simulink model "ALFlight3"  (R2019a)
settings: Solver=VariableStepAuto  StartTime=0.0  StopTime=100  RelTol=1e-3
InitFcn:
  | Ts=.05
  | load('goodMPC.mat')
  | %load('fault2mpc.mat')
  | global counts
  | counts=0
  | 
  | An=[-0.0220400000000000,0.00142200000000000,0,-32.1700000000000,0,0,0,0,0,0;-0.0575900000000000,-0.394300000000000,871,0,0,0,0,0,0,0;-9.50000000000000e-05,-0.00179300000000000,-0.546800000000000,0,0,0,0,0,0,0;0,0,1,0,0,0,0,0,0,0;0,0,0,0,-0.0639900000000000,0,-1,0.0369100000000000,0,0;0,0,0,0,-2.11100000000000,-0.504800000000000,0.193000000000000,0,0,0;0,0,0,0,0.773200000000000,0.0108700000000000,-0.179400000000000,0,0,0;0,0,0,0,0,1,0,0,0,0;0,0,0,0,0,0,1,0,0,0;0,1,0,0,0,0,0,0,0,0]
  | Bn=[0,1.91000000000000e-05,0,0;-18.5800000000000,0,0,0;-1.20000000000000,0,0,0;0,0,0,0;0,0,0,0.00839000000000000;0,0,0.184800000000000,0.105600000000000;0,0,-0.00869900000000000,-0.459100000000000;0,0,0,0;0,0,0,0;0,0,0,0]
  | 
  | load('finalWorkspace.mat')
  |  set_param('ALFlight3/ConstantA','Value','An')
  |  set_param('ALFlight3/ConstantB','Value','Bn')
model workspace (MAT data in the model file):
  Uncertainty = Simulink.Signal
  Uncertainty.DataType = 'double'
  Uncertainty.Dimensions = -1
  Uncertainty.DimensionsMode = 'auto'
  Uncertainty.Complexity = 'auto'
  Uncertainty.SampleTime = -1
  Uncertainty.SamplingMode = 'auto'
  Uncertainty.InitialValue = '10000'
values from neighbouring files (symbols this model uses):
  AfU = [-0.0194355650403 0 0.00129160400584 0 0 0 0 0 0 0 0.0910789295705 -0.529233298764 ... (100 elements, 10x10)]    [finalWorkspace.mat]
  BfU = [0 -0.0292332987635 -0.465820206007 0 0 0 0 0 0 0 4.775e-06 0 ... (40 elements, 10x4)]    [finalWorkspace.mat]
  Cn = [1 0 0 0 0 0 0 0 0 0 0 0 ... (40 elements, 4x10)]    [UpdatedWorkspace.mat]    (also in current2.mat; finalWorkspace.mat)
  Dn = [0 0 0 0 0 0 0 0 0 0 0 0 ... (16 elements, 4x4)]    [UpdatedWorkspace.mat]    (also in current2.mat; finalWorkspace.mat)
  p = 15    [calcVar.m]    (also in chanceConstraintProgramming4.m = [norminv(.505),norminv(.6),norminv(.7),norminv(.8),norminv(.; dynamicsEst.m)
undefined symbols (not defined in the file or in its folder): Earth, iA, lastPcov, lastu, lastx, MDscale, MVscale, nCC, nu, nud, nv, ny, nym, RMVscale, RYscale, ts, uoff, WGS84, xoff, Yscale
libraries: mpcsigdimcheck_private x26, simulink_extras x3, aerolibtransform2 x1, aerolibfltsims x1, commchan3 x1, aerolibanimutils x1
(part 1 of 2)
settings Model: OrderedModelArguments=off  Creator=mschr  LastModifiedBy=mschr

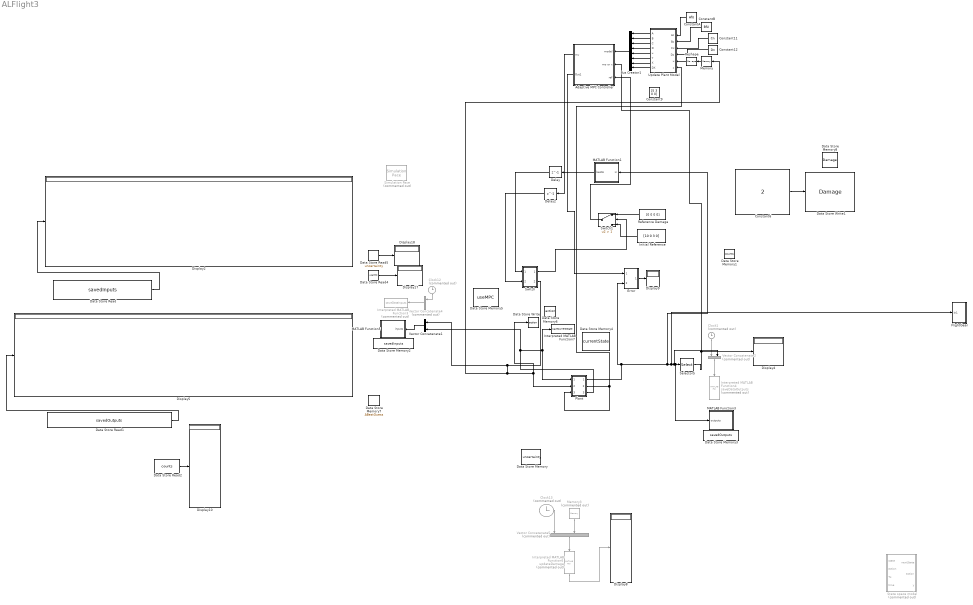
== system ALFlight3 ==
  Adaptive MPC Controller : Subsystem  AncestorBlock=mpclib/Adaptive MPC Controller  SCDEnableBlockLinearizationSpecification=on  InitFcn=ampcblock_InitFcn  StartFcn=ampcblock_StartFcn  mask(Adaptive MPC){mpcobj=mpcNominalAdaptive, x0=, enable_value=0, updateMPCinCallerWorkspace=on, md_inport=off, mv_inport=off, uref_inport=off, return_cost=off, return_mvseq=off, return_qpstatus=off, return_xseq=off, return_state=off, return_ovseq=off, state_inport=off, isltv_plant=off, umin_inport=off, umax_inport=off, ymin_inport=off, ymax_inport=off, cc_inport=off, ywt_inport=off, uwt_inport=off, duwt_inport=off, rhoeps_inport=off, pm_inport=off, MaximumP=10, HorizonChoice=FixedHorizon, BlockDataType=double, SampleTimeInherited=off, switch_inport=off}
      mask prompts: mpcobj "MPC:general:BlgAMPC"; x0 "MPC:general:BlgState"; enable_value "Value enabling optimization"; updateMPCinCallerWorkspace "Update MPC object in caller workspace"; md_inport "MPC:general:BlgMD"; mv_inport "MPC:general:BlgEXTMV"; uref_inport "MPC:general:BlgMVTARGET"; return_cost "MPC:general:BlgCOST"; return_mvseq "MPC:general:BlgMVSEQ"; return_qpstatus "MPC:general:BlgQPSTATUS"; return_xseq "MPC:general:BlgXSEQ"; return_state "MPC:general:BlgESTSTATE"; return_ovseq "MPC:general:BlgOVSEQ"; state_inport "MPC:general:BlgXKK"; isltv_plant "MPC:general:BlgLTV"; umin_inport "MPC:general:BlgMVMin"; umax_inport "MPC:general:BlgMVMax"; ymin_inport "MPC:general:BlgOVMin"; ymax_inport "MPC:general:BlgOVMax"; cc_inport "Custom constraints (E, F, G, S)"; ywt_inport "MPC:general:BlgYWT"; uwt_inport "MPC:general:BlgUWT"; duwt_inport "MPC:general:BlgDUWT"; rhoeps_inport "MPC:general:BlgECRWT"; pm_inport "MPC:general:BlgPM"; MaximumP "MPC:general:BlgMaximumP"; HorizonChoice "Simulink:Variants:LabelComboBox"; BlockDataType "MPC:general:BlgDATATYPE"; SampleTimeInherited "MPC:general:BlgTS"; switch_inport "MPC:general:BlgSWITCH"
      mask help: MPC:utility:MaskDescAdaptiveMPC1
      mask init:
      | [blk,ts,A,B,C,D,isQP,strmoorx,nmoorx,nu,nv,ny,nx,nym,nud,...
      |     degrees,lastPcov,H,Hinv,Linv,iA,Ac,Kx,Ku1,Kut,Kr,Kv,...
      |     Mlim,Mx,Mu1,Mv,z_degrees,utarget,...
      |     lastx,lastu,p,xoff,uoff,yoff,voff,myoff,no_md,no_ref,...
      |     maxiter,CustomSolver,CustomSolverCodeGen,UseWarmStart,UseSuboptimalSolution,...
      |     nxQP,openloopflag,no_ym,no_mv,no_uref,...
      |     no_umin,no_umax,no_ymin,no_ymax,no_cc,...
      |     no_switch,CustomEstimation,...
      |     no_ywt, no_uwt, no_duwt, no_rhoeps,...
      |     Wy,Wdu,Jm,SuJm,Su1,Sx,Hv,Wu,I1,...
      |     isAdaptive, isLTV, Mrows, nCC, Ecc, Fcc, Scc, Gcc, Cid, Did, ...
      |     nxp, nup, nxid, mvindex, mdindex, unindex, myindex, ...
      |     Uscale, Yscale, MVscale, MDscale, ...
      |     RYscale,RMYscale,RMVscale,RMDscale,no_p,no_m,p0] = ampcblock_MaskInitFcnParameter();
      | ampcblock_MaskInitFcnResize(gcb,nv,nu,ny,nCC);
      mask Help: eval('mpcCSHelp(''MPCmaskAdaptive'',''HelpBrowser'')');
      mask Callback pm_inport: mpcblocks_callbackPM(gcb);
      mask TypeOptions HorizonChoice: MPC/optimizer/LabelModeActiveChoice
      mask DialogControl mpcobj Prompt: Adaptive MPC Controller
      mask DialogControl x0 Prompt: Initial Controller State
      mask DialogControl Container5 Prompt: MPC:general:BlgTab1
      mask DialogControl Container6 Prompt: MPC:general:BlgBox11
      mask DialogControl md_inport Prompt: Measured disturbance (md)
      mask DialogControl mv_inport Prompt: External manipulated variable (ext.mv)
      mask DialogControl uref_inport Prompt: Targets for manipulated variables (mv.target)
      mask DialogControl Container7 Prompt: MPC:general:BlgBox12
      mask DialogControl return_cost Prompt: Optimal cost (cost)
      mask DialogControl return_mvseq Prompt: Optimal control sequence (mv.seq)
      mask DialogControl return_qpstatus Prompt: Optimization status (qp.status)
      mask DialogControl return_xseq Prompt: Optimal state sequence (x.seq)
      mask DialogControl return_state Prompt: Estimated controller states (est.state)
      mask DialogControl return_ovseq Prompt: Optimal output sequence (y.seq)
      mask DialogControl Container16 Prompt: MPC:general:BlgBox13
      mask DialogControl state_inport Prompt: Use custom state estimation instead of using the built-in Kalman filter (x[k|k])
      mask DialogControl Container9 Prompt: MPC:general:BlgTab2
      mask DialogControl Container19 Prompt: MPC:general:BlgBox20
      mask DialogControl isltv_plant Prompt: Linear Time-Varying (LTV) plants (model expects 3-D signals)
      mask DialogControl Container10 Prompt: MPC:general:BlgBox21
      mask DialogControl umin_inport Prompt: Lower MV limits (umin)
      mask DialogControl umax_inport Prompt: Upper MV limits (umax)
      mask DialogControl ymin_inport Prompt: Lower OV limits (ymin)
      mask DialogControl ymax_inport Prompt: Upper OV limits (ymax)
      mask DialogControl Container11 Prompt: MPC:general:BlgBox22
      mask DialogControl ywt_inport Prompt: OV weights (y.wt)
      mask DialogControl uwt_inport Prompt: MV weights (u.wt)
      mask DialogControl duwt_inport Prompt: MVRate weights (du.wt)
      mask DialogControl rhoeps_inport Prompt: Slack variable weight (ecr.wt)
      mask DialogControl Container17 Prompt: Prediction and Control Horizons
      mask DialogControl pm_inport Prompt: Adjust prediction horizon (p) and control horizon (m) at run time
      mask DialogControl MaximumP Prompt: Maximum prediction horizon
      mask DialogControl HorizonChoice Prompt: Label mode active choice:
      mask DialogControl Container13 Prompt: MPC:general:BlgTab3
      mask DialogControl Container14 Prompt: MPC:general:BlgBox31
      mask DialogControl BlockDataType Prompt: Block Data Type
      mask DialogControl Container15 Prompt: MPC:general:BlgBox32
      mask DialogControl SampleTimeInherited Prompt: Inherit sample time (must be the same as controller sample time)
      mask DialogControl Container18 Prompt: MPC:general:BlgBox33
      mask DialogControl switch_inport Prompt: Use external signal to enable or disable optimization (switch)
      mask Display:
      | fprintf('Adaptive\nMPC');
      | port_label('output', 1, 'mv')
      | port_label('input', 1, 'model')
      | port_label('input', 2, 'mo')
      | port_label('input', 3, 'ref')
  Bus Creator1 : BusCreator  Inputs=8
  Clock1 : Clock  Commented=on
  Clock12 : Clock  Commented=on
  Clock13 : Clock  Commented=on
  Constant11 : Constant  Value=Cn
  Constant12 : Constant  Value=Dn
  Constant6 : Constant  Value=2
  Constant9 : Constant  Value=[5 3 0 0]
  ConstantA : Constant  Value=AfU
  ConstantB : Constant  Value=BfU
  Data Store Memory : DataStoreMemory  DataStoreName=uncertainty  ReadBeforeWriteMsg=warning  WriteAfterWriteMsg=warning  WriteAfterReadMsg=warning  InitialValue=10000  ShowAdditionalParam=off  OutDataTypeStr=double
  Data Store Memory1 : DataStoreMemory  DataStoreName=counts  ReadBeforeWriteMsg=warning  WriteAfterWriteMsg=warning  WriteAfterReadMsg=warning  ShowAdditionalParam=off  OutDataTypeStr=double
  Data Store Memory2 : DataStoreMemory  DataStoreName=savedInputs  ReadBeforeWriteMsg=warning  WriteAfterWriteMsg=warning  WriteAfterReadMsg=warning  InitialValue=zeros(15,5000)  ShowAdditionalParam=off  OutDataTypeStr=double
  Data Store Memory3 : DataStoreMemory  DataStoreName=savedOutputs  ReadBeforeWriteMsg=warning  WriteAfterWriteMsg=warning  WriteAfterReadMsg=warning  InitialValue=zeros(11,5000)  ShowAdditionalParam=off  OutDataTypeStr=double
  Data Store Memory4 : DataStoreMemory  DataStoreName=currentState  ReadBeforeWriteMsg=warning  WriteAfterWriteMsg=warning  WriteAfterReadMsg=warning  InitialValue=zeros(11,1)  ShowAdditionalParam=off  OutDataTypeStr=double
  Data Store Memory5 : DataStoreMemory  DataStoreName=useMPC  ReadBeforeWriteMsg=warning  WriteAfterWriteMsg=warning  WriteAfterReadMsg=warning  InitialValue=false  ShowAdditionalParam=off  OutDataTypeStr=boolean
  Data Store Memory6 : DataStoreMemory  DataStoreName=action  ReadBeforeWriteMsg=warning  WriteAfterWriteMsg=warning  WriteAfterReadMsg=warning  InitialValue=[0 0 0 0]  ShowAdditionalParam=off  OutDataTypeStr=double
  Data Store Memory7 : DataStoreMemory  DataStoreName=ABestGuess  ReadBeforeWriteMsg=warning  WriteAfterWriteMsg=warning  WriteAfterReadMsg=warning  InitialValue=zeros(15,11)  ShowAdditionalParam=off  OutDataTypeStr=double
  Data Store Memory8 : DataStoreMemory  DataStoreName=Damage  ReadBeforeWriteMsg=warning  WriteAfterWriteMsg=warning  WriteAfterReadMsg=warning  InitialValue=2  ShowAdditionalParam=off  OutDataTypeStr=double
  Data Store Read : DataStoreRead  DataStoreName=savedInputs
  Data Store Read1 : DataStoreRead  DataStoreName=savedOutputs
  Data Store Read2 : DataStoreRead  DataStoreName=counts
  Data Store Read4 : DataStoreRead  DataStoreName=useMPC
  Data Store Read5 : DataStoreRead  DataStoreName=uncertainty
  Data Store Write : DataStoreWrite  DataStoreName=action
  Data Store Write1 : DataStoreWrite  DataStoreName=Damage
  Delay : Delay  DelayLength=1  InitialCondition=0
  Delay2 : Delay  DelayLength=1  InitialCondition=0
  Display{2,4..5,8..10,17..18} (8 alike) : Display
  Error : Subsystem
  FlightGear : Subsystem
  Initial Reference : Constant  Value=[10 0 3 0]
  Interpreted MATLAB Function3 : MATLABFcn  Commented=on  MATLABFcn=saveDataInputs  OutputDimensions=0
  Interpreted MATLAB Function4 : MATLABFcn  Commented=on  MATLABFcn=saveDataOutputs  OutputDimensions=0
  Interpreted MATLAB Function6 : MATLABFcn  Commented=on  MATLABFcn=updateDamage  OutputDimensions=4
  Interpreted MATLAB Function7 : MATLABFcn  MATLABFcn=saveCurrentState  OutputDimensions=0
  MATLAB Function1 : MATLAB Function  TreatAsAtomicUnit=on
      settings: MinAlgLoopOccurrences=on
  MATLAB Function3 : MATLAB Function  TreatAsAtomicUnit=on
  MATLAB Function5 : MATLAB Function  TreatAsAtomicUnit=on
  Memory : Memory  InitialCondition=zeros(4,1)
  Memory3 : Memory  Commented=on  InitialCondition=zeros(11,1)  InheritSampleTime=on
  Plant : Subsystem
  Reference Damage : Constant  Value=[0 0 0 0]
  Reshape : Reshape  OutputDimensionality=Customize  OutputDimensions=[4,1]
  Selector5 : Selector  InputPortWidth=11  IndexOptions=Index vector (dialog)  Indices=[1 8 9 11]  OutputSizes=1
  Simulation Pace : aerolibanimutils/Simulation Pace  Commented=on  SimulationPace=1  SleepMode=Auto  OutputPaceError=off  SampleTime=1/30
  State space model : MATLAB Function  Commented=on  TreatAsAtomicUnit=on  SystemSampleTime=.05
      settings: MinAlgLoopOccurrences=on
  "Switch " : Subsystem
  Switch1 : Switch  Criteria=u2 > Threshold  Threshold=1
  Update Plant Model : MATLAB Function  TreatAsAtomicUnit=on
  Vector Concatenate1 : Concatenate
  Vector Concatenate2 : Concatenate  Commented=on
  Vector Concatenate4 : Concatenate  Commented=on  NumInputs=3
  Vector Concatenate5 : Concatenate  Commented=on  NumInputs=4
  wires:
  Vector Concatenate2/1 -> Interpreted MATLAB Function4/1
  Clock1/1 -> Vector Concatenate2/1
  Reference Damage/1 -> Switch1/1
  Vector Concatenate4/1 -> Interpreted MATLAB Function3/1
  Clock12/1 -> Vector Concatenate4/1
  Vector Concatenate5/1 -> Interpreted MATLAB Function6/1
  Memory3/1 -> Vector Concatenate5/3
  Clock13/1 -> Vector Concatenate5/1
  Interpreted MATLAB Function6/1 -> Display8/1
  MATLAB Function1/1(bestA) -> Delay/1
  Vector Concatenate1/1 -> MATLAB Function5/1(inputs)
  Adaptive MPC Controller/1(mv) -> Delay2/1
  Data Store Read/1 -> Display2/1
  Data Store Read1/1 -> Display5/1
  Data Store Read2/1 -> Display10/1
  Delay2/1 -> "Switch "/2(In2)
  Adaptive MPC Controller/2(Out1) -> Error/1(In1)
  Data Store Read4/1 -> Display17/1
  Data Store Read5/1 -> Display18/1
  Initial Reference/1 -> Switch1/3
  Switch1/1 -> Adaptive MPC Controller/3(ref)
  Memory/1 -> Reshape/1
  Update Plant Model/7(X) -> Bus Creator1/7
  Update Plant Model/8(DX) -> Bus Creator1/8
  Update Plant Model/6(Y) -> Bus Creator1/6
  Update Plant Model/3(C) -> Bus Creator1/3
  Update Plant Model/1(A) -> Bus Creator1/1
  Update Plant Model/4(D) -> Bus Creator1/4
  Update Plant Model/2(B) -> Bus Creator1/2
  Reshape/1 -> Update Plant Model/5("u ")
  Constant12/1 -> Update Plant Model/4(Dc)
  ConstantB/1 -> Update Plant Model/2(Bc)
  Constant11/1 -> Update Plant Model/3(Cc)
  ConstantA/1 -> Update Plant Model/1(Ac)
  Selector5/1 -> Adaptive MPC Controller/2(mo or x), Display4/1
  Bus Creator1/1 -> Adaptive MPC Controller/1(model)
  Update Plant Model/5(u) -> Bus Creator1/5
  Constant6/1 -> Data Store Write1/1
  Plant/3(Out3) -> Vector Concatenate1/2, Plant/1(In1), Interpreted MATLAB Function7/1
  Plant/2(Out2) -> Update Plant Model/6(x), Plant/3(In3)
  Plant/1(Out1) -> MATLAB Function1/1(in), FlightGear/1(In1), Vector Concatenate2/2, MATLAB Function3/1(outputs), Selector5/1, Error/2(In2)
  "Switch "/2(Out2) -> Vector Concatenate1/1, Memory/1, Plant/2(In2), Data Store Write/1
  Delay/1 -> "Switch "/1(In1)
  "Switch "/1(Out1) -> Switch1/2
  Error/1(Out1) -> Display9/1

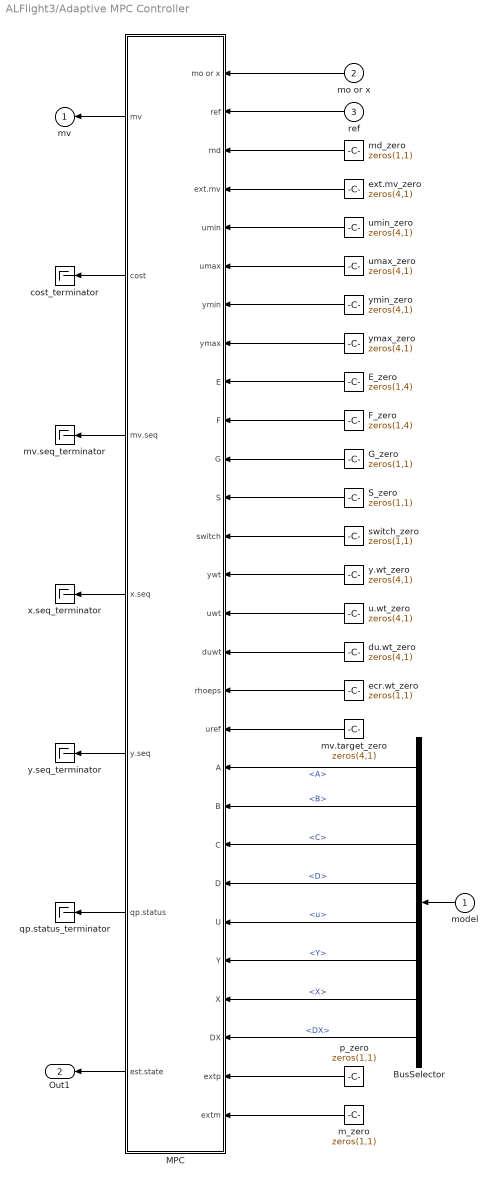
== system ALFlight3/Adaptive MPC Controller ==
  model : Inport
  mo or x : Inport  Port=2
  ref : Inport  Port=3
  BusSelector : BusSelector  OutputSignals=A,B,C,D,u,Y,X,DX
  E_zero : Constant  Value=zeros(1,4)  VectorParams1D=off  OutDataTypeStr=BlockDataType
  F_zero : Constant  Value=zeros(1,4)  VectorParams1D=off  OutDataTypeStr=BlockDataType
  G_zero : Constant  Value=zeros(1,1)  VectorParams1D=off  OutDataTypeStr=BlockDataType
  MPC : Subsystem
  S_zero : Constant  Value=zeros(1,1)  VectorParams1D=off  OutDataTypeStr=BlockDataType
  cost_terminator : Terminator
  du.wt_zero : Constant  Value=zeros(4,1)  OutDataTypeStr=BlockDataType
  ecr.wt_zero : Constant  Value=zeros(1,1)  OutDataTypeStr=BlockDataType
  ext.mv_zero : Constant  Value=zeros(4,1)  OutDataTypeStr=BlockDataType
  m_zero : Constant  Value=zeros(1,1)  OutDataTypeStr=BlockDataType
  md_zero : Constant  Value=zeros(1,1)  OutDataTypeStr=BlockDataType
  mv.seq_terminator : Terminator
  mv.target_zero : Constant  Value=zeros(4,1)  OutDataTypeStr=BlockDataType
  p_zero : Constant  Value=zeros(1,1)  OutDataTypeStr=BlockDataType
  qp.status_terminator : Terminator
  switch_zero : Constant  Value=zeros(1,1)  OutDataTypeStr=BlockDataType
  u.wt_zero : Constant  Value=zeros(4,1)  OutDataTypeStr=BlockDataType
  umax_zero : Constant  Value=zeros(4,1)  OutDataTypeStr=BlockDataType
  umin_zero : Constant  Value=zeros(4,1)  OutDataTypeStr=BlockDataType
  x.seq_terminator : Terminator
  y.seq_terminator : Terminator
  y.wt_zero : Constant  Value=zeros(4,1)  OutDataTypeStr=BlockDataType
  ymax_zero : Constant  Value=zeros(4,1)  OutDataTypeStr=BlockDataType
  ymin_zero : Constant  Value=zeros(4,1)  OutDataTypeStr=BlockDataType
  mv : Outport
  Out1 : Outport  Port=2
  wires:
  m_zero/1 -> MPC/28(extm)
  p_zero/1 -> MPC/27(extp)
  MPC/5(y.seq) -> y.seq_terminator/1
  MPC/4(x.seq) -> x.seq_terminator/1
  G_zero/1 -> MPC/11(G)
  F_zero/1 -> MPC/10(F)
  E_zero/1 -> MPC/9(E)
  S_zero/1 -> MPC/12(S)
  MPC/7(est.state) -> Out1/1
  y.wt_zero/1 -> MPC/14(ywt)
  switch_zero/1 -> MPC/13(switch)
  ymin_zero/1 -> MPC/7(ymin)
  umax_zero/1 -> MPC/6(umax)
  umin_zero/1 -> MPC/5(umin)
  u.wt_zero/1 -> MPC/15(uwt)
  ymax_zero/1 -> MPC/8(ymax)
  du.wt_zero/1 -> MPC/16(duwt)
  ecr.wt_zero/1 -> MPC/17(rhoeps)
  mv.target_zero/1 -> MPC/18(uref)
  ext.mv_zero/1 -> MPC/4(ext.mv)
  BusSelector/8 -> MPC/26(DX)  "<DX>"
  BusSelector/7 -> MPC/25(X)  "<X>"
  BusSelector/6 -> MPC/24(Y)  "<Y>"
  BusSelector/5 -> MPC/23(U)  "<u>"
  model/1 -> BusSelector/1
  BusSelector/4 -> MPC/22(D)  "<D>"
  BusSelector/3 -> MPC/21(C)  "<C>"
  BusSelector/2 -> MPC/20(B)  "<B>"
  BusSelector/1 -> MPC/19(A)  "<A>"
  MPC/6(qp.status) -> qp.status_terminator/1
  MPC/3(mv.seq) -> mv.seq_terminator/1
  MPC/2(cost) -> cost_terminator/1
  ref/1 -> MPC/2(ref)
  mo or x/1 -> MPC/1(mo or x)
  MPC/1(mv) -> mv/1
  md_zero/1 -> MPC/3(md)

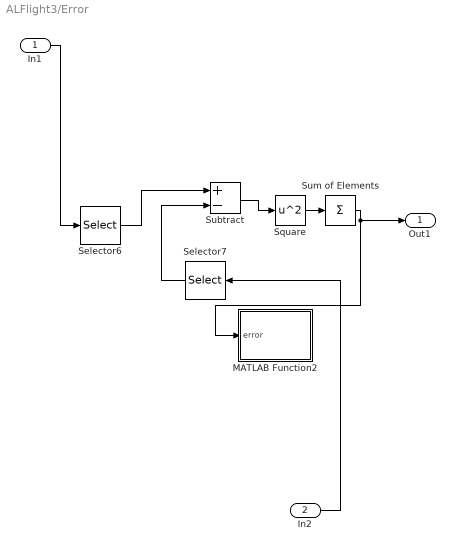
== system ALFlight3/Error ==
  In1 : Inport
  In2 : Inport  Port=2
  MATLAB Function2 : MATLAB Function  TreatAsAtomicUnit=on
  Selector6 : Selector  InputPortWidth=12  IndexOptions=Index vector (dialog)  Indices=[1 2 3 4 5 6 7 8 9]  OutputSizes=1
  Selector7 : Selector  InputPortWidth=11  IndexOptions=Index vector (dialog)  Indices=[1 2 3 4 5 6 7 8 9]  OutputSizes=1
  Square : Math  Operator=square  SaturateOnIntegerOverflow=on
  Subtract : Sum  Inputs=+-
  Sum of Elements : Sum  Inputs=+
  Out1 : Outport
  wires:
  Square/1 -> Sum of Elements/1
  Selector6/1 -> Subtract/1
  Sum of Elements/1 -> Out1/1, MATLAB Function2/1(error)
  Selector7/1 -> Subtract/2
  Subtract/1 -> Square/1
  In1/1 -> Selector6/1
  In2/1 -> Selector7/1

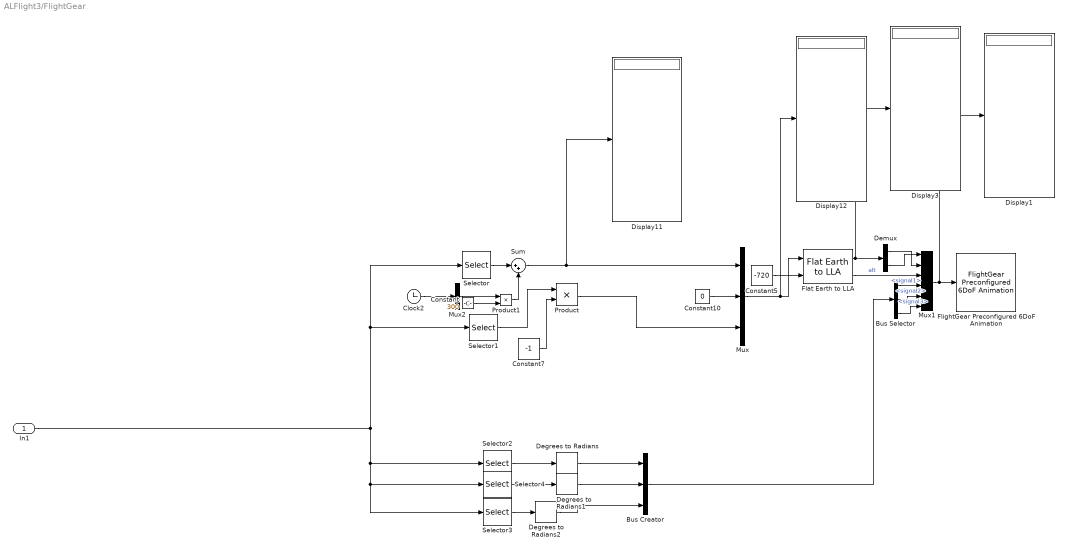
== system ALFlight3/FlightGear ==
  In1 : Inport
  Bus Creator : BusCreator  Inputs=3
  Bus Selector : BusSelector  OutputSignals=signal1,signal2,signal3
  Clock2 : Clock
  Constant : Constant  Value=300  SampleTime=.05
  Constant10 : Constant  Value=0
  Constant5 : Constant  Value=-720
  Constant7 : Constant  Value=-1
  Degrees to Radians : simulink_extras/Transformations/Degrees to Radians
  Degrees to Radians1 : simulink_extras/Transformations/Degrees to Radians
  Degrees to Radians2 : simulink_extras/Transformations/Degrees to Radians
  Demux : Demux  Outputs=2
  Display{1,3,11..12} (4 alike) : Display
  Flat Earth to LLA : aerolibtransform2/Flat Earth to LLA  units=English  ptype=Earth (WGS84)  F=1/298.257223563  R=20925646.3255  LL0=[21.31835828 -157.9232806]  psi=0
  FlightGear Preconfigured 6DoF Animation : aerolibfltsims/FlightGear Preconfigured 6DoF Animation  xFlightGearVersion=v2018.2  DestinationIpAddress=127.0.0.1  DestinationPort=5502  SampleTime=.05  packetVersion=24
      settings: SourceProductName=Aerospace Blockset
  Mux : Mux  Inputs=3
  Mux1 : Mux  Inputs=6
  Mux2 : Mux  Inputs=1
  Product : Product
  Product1 : Product
  Selector : Selector  InputPortWidth=11  IndexOptions=Index vector (dialog)  Indices=10  OutputSizes=1
  Selector1 : Selector  InputPortWidth=11  IndexOptions=Index vector (dialog)  Indices=11  OutputSizes=1
  Selector2 : Selector  InputPortWidth=11  IndexOptions=Index vector (dialog)  Indices=8  OutputSizes=1
  Selector3 : Selector  InputPortWidth=11  IndexOptions=Index vector (dialog)  Indices=9  OutputSizes=1
  Selector4 : Selector  InputPortWidth=11  IndexOptions=Index vector (dialog)  Indices=4  OutputSizes=1
  Sum : Sum  Inputs=|++
  wires:
  Constant10/1 -> Mux/2
  Product/1 -> Mux/3
  Bus Selector/1 -> Mux1/4  "<signal1>"
  Flat Earth to LLA/1 -> Display3/1, Demux/1
  Sum/1 -> Display11/1, Mux/1
  Demux/2 -> Mux1/1
  In1/1 -> Selector1/1, Selector/1, Selector2/1, Selector4/1, Selector3/1
  Mux/1 -> Flat Earth to LLA/1, Display12/1
  Clock2/1 -> Mux2/1
  Degrees to Radians/1 -> Bus Creator/1
  Bus Selector/2 -> Mux1/5  "<signal2>"
  Constant7/1 -> Product/2
  Constant/1 -> Product1/2
  Bus Selector/3 -> Mux1/6  "<signal3>"
  Selector/1 -> Sum/1
  Selector3/1 -> Degrees to Radians2/1
  Degrees to Radians1/1 -> Bus Creator/2
  Demux/1 -> Mux1/2
  Constant5/1 -> Flat Earth to LLA/2
  Product1/1 -> Sum/2
  Mux2/1 -> Product1/1
  Selector2/1 -> Degrees to Radians/1
  Bus Creator/1 -> Bus Selector/1
  Degrees to Radians2/1 -> Bus Creator/3
  Selector1/1 -> Product/1
  Mux1/1 -> Display1/1, FlightGear Preconfigured 6DoF Animation/1
  Flat Earth to LLA/2 -> Mux1/3  "alt"
  Selector4/1 -> Degrees to Radians1/1

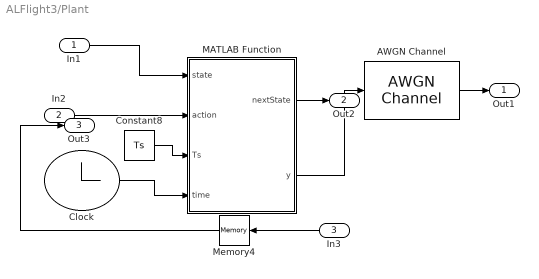
== system ALFlight3/Plant ==
  In1 : Inport
  In2 : Inport  Port=2
  In3 : Inport  Port=3
  AWGN Channel : commchan3/AWGN Channel  InputProcessing=Columns as channels (frame based)  seed=90  noiseMode="Signal to noise ratio  (SNR)"  EbNodB=50  EsNodB=10  SNRdB=100  bitsPerSym=1  Ps=1  Tsym=1  variance=1
      settings: SourceProductName=Communications Toolbox
  Clock : Clock
  Constant8 : Constant  Value=Ts
  MATLAB Function : MATLAB Function  TreatAsAtomicUnit=on  SystemSampleTime=.05
      settings: MinAlgLoopOccurrences=on
  Memory4 : Memory  InitialCondition=zeros(11,1)  InheritSampleTime=on  LinearizeAsDelay=on
  Out1 : Outport
  Out2 : Outport  Port=2
  Out3 : Outport  Port=3
  wires:
  Memory4/1 -> Out3/1
  AWGN Channel/1 -> Out1/1
  Constant8/1 -> MATLAB Function/3(Ts)
  In3/1 -> Memory4/1
  MATLAB Function/1(nextState) -> Out2/1
  Clock/1 -> MATLAB Function/4(time)
  MATLAB Function/2(y) -> AWGN Channel/1
  In2/1 -> MATLAB Function/2(action)
  In1/1 -> MATLAB Function/1(state)

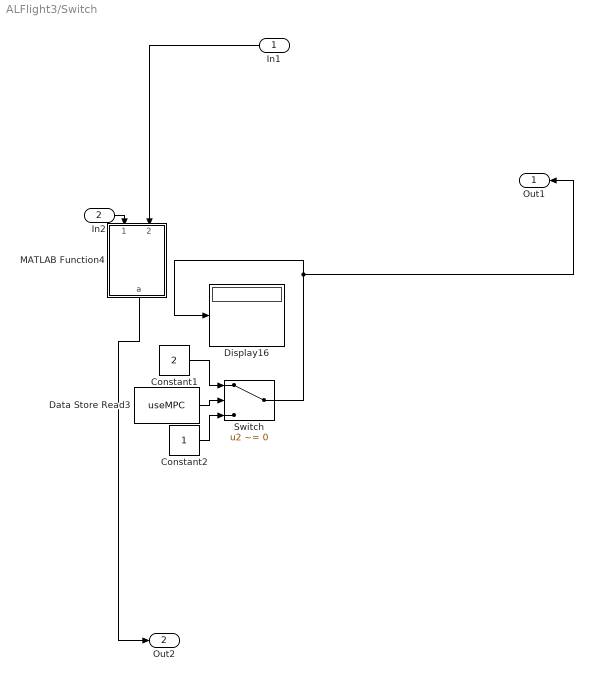
== system ALFlight3/Switch  ==
  In1 : Inport
  In2 : Inport  Port=2
  Constant1 : Constant  Value=2
  Constant2 : Constant
  Data Store Read3 : DataStoreRead  DataStoreName=useMPC
  Display16 : Display
  MATLAB Function4 : MATLAB Function  TreatAsAtomicUnit=on  SystemSampleTime=.05
      settings: MinAlgLoopOccurrences=on
  Switch : Switch  Criteria=u2 ~= 0  Threshold=.01
  Out1 : Outport
  Out2 : Outport  Port=2
  wires:
  Constant2/1 -> Switch/3
  In1/1 -> MATLAB Function4/2(actionAL)
  Switch/1 -> Out1/1, Display16/1
  Data Store Read3/1 -> Switch/2
  MATLAB Function4/1(a) -> Out2/1
  Constant1/1 -> Switch/1
  In2/1 -> MATLAB Function4/1(actionMPC)

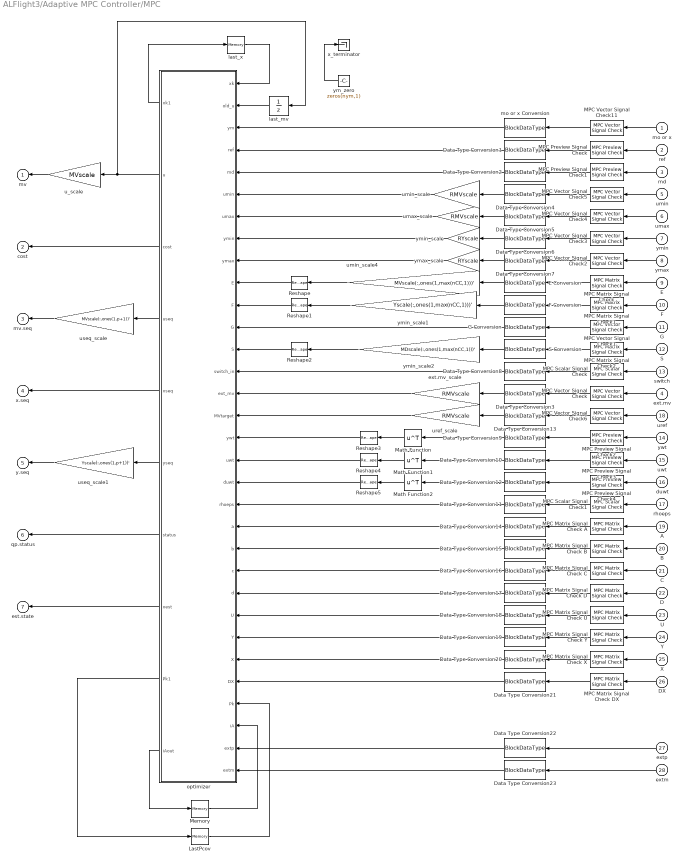
== system ALFlight3/Adaptive MPC Controller/MPC ==
  mo or x : Inport
  ref : Inport  Port=2
  md : Inport  Port=3
  ext.mv : Inport  Port=4
  umin : Inport  Port=5
  umax : Inport  Port=6
  ymin : Inport  Port=7
  ymax : Inport  Port=8
  E : Inport  Port=9
  F : Inport  Port=10
  G : Inport  Port=11
  S : Inport  Port=12
  switch : Inport  Port=13
  ywt : Inport  Port=14
  uwt : Inport  Port=15
  duwt : Inport  Port=16
  rhoeps : Inport  Port=17
  uref : Inport  Port=18
  A : Inport  Port=19
  B : Inport  Port=20
  C : Inport  Port=21
  D : Inport  Port=22
  U : Inport  Port=23
  Y : Inport  Port=24
  X : Inport  Port=25
  DX : Inport  Port=26
  extp : Inport  Port=27
  extm : Inport  Port=28
  Data Type Conversion{1..23} (23 alike) : DataTypeConversion  OutDataTypeStr=BlockDataType
  E Conversion : DataTypeConversion  OutDataTypeStr=BlockDataType
  F Conversion : DataTypeConversion  OutDataTypeStr=BlockDataType
  G Conversion : DataTypeConversion  OutDataTypeStr=BlockDataType
  LastPcov : Memory  InitialCondition=lastPcov  InheritSampleTime=on  LinearizeAsDelay=on
  MPC Matrix Signal Check : mpcsigdimcheck_private/MPC Matrix Signal Check  blockname=blk  signalname='CustomConstraint.E'  numrow=max(nCC,1)  numcol=nu  steps=0  isLTV=0
      settings: SourceProductName=MATLAB Runtime - Model Predictive Control Toolbox Addin  SourceProductBaseCode=Missing
  MPC Matrix Signal Check A : mpcsigdimcheck_private/MPC Matrix Signal Check  blockname=blk  signalname='Model.A'  numrow=nxp  numcol=nxp  steps=p  isLTV=isLTV
      settings: SourceProductName=MATLAB Runtime - Model Predictive Control Toolbox Addin  SourceProductBaseCode=Missing
  MPC Matrix Signal Check B : mpcsigdimcheck_private/MPC Matrix Signal Check  blockname=blk  signalname='Model.B'  numrow=nxp  numcol=nu+nv-1+nud  steps=p  isLTV=isLTV
      settings: SourceProductName=MATLAB Runtime - Model Predictive Control Toolbox Addin  SourceProductBaseCode=Missing
  MPC Matrix Signal Check C : mpcsigdimcheck_private/MPC Matrix Signal Check  blockname=blk  signalname='Model.C'  numrow=ny  numcol=nxp  steps=p  isLTV=isLTV
      settings: SourceProductName=MATLAB Runtime - Model Predictive Control Toolbox Addin  SourceProductBaseCode=Missing
  MPC Matrix Signal Check D : mpcsigdimcheck_private/MPC Matrix Signal Check  blockname=blk  signalname='Model.D'  numrow=ny  numcol=nu+nv-1+nud  steps=p  isLTV=isLTV
      settings: SourceProductName=MATLAB Runtime - Model Predictive Control Toolbox Addin  SourceProductBaseCode=Missing
  MPC Matrix Signal Check DX : mpcsigdimcheck_private/MPC Matrix Signal Check  blockname=blk  signalname='Model.DX'  numrow=nxp  numcol=1  steps=p  isLTV=isLTV
      settings: SourceProductName=MATLAB Runtime - Model Predictive Control Toolbox Addin  SourceProductBaseCode=Missing
  MPC Matrix Signal Check U : mpcsigdimcheck_private/MPC Matrix Signal Check  blockname=blk  signalname='Model.U'  numrow=nu+nv-1+nud  numcol=1  steps=p  isLTV=isLTV
      settings: SourceProductName=MATLAB Runtime - Model Predictive Control Toolbox Addin  SourceProductBaseCode=Missing
  MPC Matrix Signal Check X : mpcsigdimcheck_private/MPC Matrix Signal Check  blockname=blk  signalname='Model.X'  numrow=nxp  numcol=1  steps=p  isLTV=isLTV
      settings: SourceProductName=MATLAB Runtime - Model Predictive Control Toolbox Addin  SourceProductBaseCode=Missing
  MPC Matrix Signal Check Y : mpcsigdimcheck_private/MPC Matrix Signal Check  blockname=blk  signalname='Model.Y'  numrow=ny  numcol=1  steps=p  isLTV=isLTV
      settings: SourceProductName=MATLAB Runtime - Model Predictive Control Toolbox Addin  SourceProductBaseCode=Missing
  MPC Matrix Signal Check1 : mpcsigdimcheck_private/MPC Matrix Signal Check  blockname=blk  signalname='CustomConstraint.F'  numrow=max(nCC,1)  numcol=ny  steps=0  isLTV=0
      settings: SourceProductName=MATLAB Runtime - Model Predictive Control Toolbox Addin  SourceProductBaseCode=Missing
  MPC Matrix Signal Check2 : mpcsigdimcheck_private/MPC Matrix Signal Check  blockname=blk  signalname='CustomConstraint.S'  numrow=max(nCC,1)  numcol=max(nv-1,1)  steps=0  isLTV=0
      settings: SourceProductName=MATLAB Runtime - Model Predictive Control Toolbox Addin  SourceProductBaseCode=Missing
  MPC Preview Signal Check : mpcsigdimcheck_private/MPC Preview Signal Check  blockname=blk  signalname='ref'  numrow=p  numcol=ny
      settings: SourceProductName=MATLAB Runtime - Model Predictive Control Toolbox Addin  SourceProductBaseCode=Missing
  MPC Preview Signal Check1 : mpcsigdimcheck_private/MPC Preview Signal Check  blockname=blk  signalname='md'  numrow=p+1  numcol=max(nv-1,1)
      settings: SourceProductName=MATLAB Runtime - Model Predictive Control Toolbox Addin  SourceProductBaseCode=Missing
  MPC Preview Signal Check2 : mpcsigdimcheck_private/MPC Preview Signal Check  blockname=blk  signalname='y.wt'  numrow=p  numcol=ny
      settings: SourceProductName=MATLAB Runtime - Model Predictive Control Toolbox Addin  SourceProductBaseCode=Missing
  MPC Preview Signal Check3 : mpcsigdimcheck_private/MPC Preview Signal Check  blockname=blk  signalname='u.wt'  numrow=p  numcol=nu
      settings: SourceProductName=MATLAB Runtime - Model Predictive Control Toolbox Addin  SourceProductBaseCode=Missing
  MPC Preview Signal Check4 : mpcsigdimcheck_private/MPC Preview Signal Check  blockname=blk  signalname='du.wt'  numrow=p  numcol=nu
      settings: SourceProductName=MATLAB Runtime - Model Predictive Control Toolbox Addin  SourceProductBaseCode=Missing
  MPC Scalar Signal Check : mpcsigdimcheck_private/MPC Scalar Signal Check  blockname=blk  signalname='switch'
      settings: SourceProductName=MATLAB Runtime - Model Predictive Control Toolbox Addin  SourceProductBaseCode=Missing
  MPC Scalar Signal Check1 : mpcsigdimcheck_private/MPC Scalar Signal Check  blockname=blk  signalname='ecr.wt'
      settings: SourceProductName=MATLAB Runtime - Model Predictive Control Toolbox Addin  SourceProductBaseCode=Missing
  MPC Vector Signal Check : mpcsigdimcheck_private/MPC Vector Signal Check  blockname=blk  signalname='ext.mv'  num=nu  vectortype=Any
      settings: SourceProductName=MATLAB Runtime - Model Predictive Control Toolbox Addin  SourceProductBaseCode=Missing
  MPC Vector Signal Check1 : mpcsigdimcheck_private/MPC Vector Signal Check  blockname=blk  signalname='CustomConstraint.G'  num=max(nCC,1)  vectortype=Column
      settings: SourceProductName=MATLAB Runtime - Model Predictive Control Toolbox Addin  SourceProductBaseCode=Missing
  MPC Vector Signal Check11 : mpcsigdimcheck_private/MPC Vector Signal Check  blockname=blk  signalname=strmoorx  num=nmoorx  vectortype=Any
      settings: SourceProductName=MATLAB Runtime - Model Predictive Control Toolbox Addin  SourceProductBaseCode=Missing
  MPC Vector Signal Check2 : mpcsigdimcheck_private/MPC Vector Signal Check  blockname=blk  signalname='ymax'  num=ny  vectortype=Any
      settings: SourceProductName=MATLAB Runtime - Model Predictive Control Toolbox Addin  SourceProductBaseCode=Missing
  MPC Vector Signal Check3 : mpcsigdimcheck_private/MPC Vector Signal Check  blockname=blk  signalname='ymin'  num=ny  vectortype=Any
      settings: SourceProductName=MATLAB Runtime - Model Predictive Control Toolbox Addin  SourceProductBaseCode=Missing
  MPC Vector Signal Check4 : mpcsigdimcheck_private/MPC Vector Signal Check  blockname=blk  signalname='umax'  num=nu  vectortype=Any
      settings: SourceProductName=MATLAB Runtime - Model Predictive Control Toolbox Addin  SourceProductBaseCode=Missing
  MPC Vector Signal Check5 : mpcsigdimcheck_private/MPC Vector Signal Check  blockname=blk  signalname='umin'  num=nu  vectortype=Any
      settings: SourceProductName=MATLAB Runtime - Model Predictive Control Toolbox Addin  SourceProductBaseCode=Missing
  MPC Vector Signal Check6 : mpcsigdimcheck_private/MPC Vector Signal Check  blockname=blk  signalname='mv.target'  num=nu  vectortype=Any
      settings: SourceProductName=MATLAB Runtime - Model Predictive Control Toolbox Addin  SourceProductBaseCode=Missing
  Math Function : Math  Operator=transpose  SaturateOnIntegerOverflow=on
  Math Function1 : Math  Operator=transpose  SaturateOnIntegerOverflow=on
  Math Function2 : Math  Operator=transpose  SaturateOnIntegerOverflow=on
  Memory : Memory  InitialCondition=iA  InheritSampleTime=on  LinearizeAsDelay=on
  Reshape : Reshape  OutputDimensionality=Customize  OutputDimensions=double([max(nCC,1),nu])
  Reshape1 : Reshape  OutputDimensionality=Customize  OutputDimensions=double([max(nCC,1),ny])
  Reshape2 : Reshape  OutputDimensionality=Customize  OutputDimensions=double([max(nCC,1),max(nv-1,1)])
  Reshape3 : Reshape  OutputDimensionality=Column vector (2-D)
  Reshape4 : Reshape  OutputDimensionality=Column vector (2-D)
  Reshape5 : Reshape  OutputDimensionality=Column vector (2-D)
  S Conversion : DataTypeConversion  OutDataTypeStr=BlockDataType
  ext.mv_scale : Gain  Gain=RMVscale  SampleTime=ts
  last_mv : UnitDelay  InitialCondition=lastu+uoff  SampleTime=ts  HasFrameUpgradeWarning=on
  last_x : Memory  InitialCondition=lastx+xoff  InheritSampleTime=on  LinearizeAsDelay=on
  mo or x Conversion : DataTypeConversion  OutDataTypeStr=BlockDataType
  optimizer : Subsystem  VariantControlMode=Label  Variant=on  VariantControl=Variant1  LabelModeActiveChoice=FixedHorizon
  u_scale : Gain  Gain=MVscale  SampleTime=ts
  umax_scale : Gain  Gain=RMVscale  SampleTime=ts
  umin_scale : Gain  Gain=RMVscale  SampleTime=ts
  umin_scale4 : Gain  Gain=MVscale(:,ones(1,max(nCC,1)))'  SampleTime=ts
  uref_scale : Gain  Gain=RMVscale  SampleTime=ts
  useq_scale : Gain  Gain=MVscale(:,ones(1,p+1))'  SampleTime=ts
  useq_scale1 : Gain  Gain=Yscale(:,ones(1,p+1))'  SampleTime=ts
  x_terminator : Terminator
  ym_zero : Constant  Value=zeros(nym,1)  OutDataTypeStr=BlockDataType
  ymax_scale : Gain  Gain=RYscale  SampleTime=ts
  ymin_scale : Gain  Gain=RYscale  SampleTime=ts
  ymin_scale1 : Gain  Gain=Yscale(:,ones(1,max(nCC,1)))'  SampleTime=ts
  ymin_scale2 : Gain  Gain=MDscale(:,ones(1,max(nCC,1)))'  SampleTime=ts
  mv : Outport  OutDataTypeStr=BlockDataType
  cost : Outport  Port=2  OutDataTypeStr=BlockDataType
  mv.seq : Outport  Port=3  OutDataTypeStr=BlockDataType
  x.seq : Outport  Port=4  OutDataTypeStr=BlockDataType
  y.seq : Outport  Port=5  OutDataTypeStr=BlockDataType
  qp.status : Outport  Port=6  OutDataTypeStr=BlockDataType
  est.state : Outport  Port=7  OutDataTypeStr=BlockDataType
  wires:
  extm/1 -> Data Type Conversion23/1
  extp/1 -> Data Type Conversion22/1
  Data Type Conversion23/1 -> optimizer/32(extm)
  Data Type Conversion22/1 -> optimizer/31(extp)
  optimizer/10(" iAout") -> Memory/1
  optimizer/9(" Pk1") -> LastPcov/1
  optimizer/8(" xest") -> est.state/1
  optimizer/7(" status") -> qp.status/1
  optimizer/6(" yseq") -> useq_scale1/1
  optimizer/5(" xseq") -> x.seq/1
  optimizer/4(" useq") -> useq_scale/1
  optimizer/3(" cost") -> cost/1
  optimizer/2(" u") -> last_mv/1, u_scale/1
  optimizer/1(" xk1") -> last_x/1
  Memory/1 -> optimizer/30("iA ")
  LastPcov/1 -> optimizer/29("Pk ")
  Data Type Conversion21/1 -> optimizer/28("DX ")
  Data Type Conversion20/1 -> optimizer/27("X ")
  Data Type Conversion19/1 -> optimizer/26("Y ")
  Data Type Conversion18/1 -> optimizer/25("U ")
  Data Type Conversion17/1 -> optimizer/24("d ")
  Data Type Conversion16/1 -> optimizer/23("c ")
  Data Type Conversion15/1 -> optimizer/22("b ")
  Data Type Conversion14/1 -> optimizer/21("a ")
  Data Type Conversion11/1 -> optimizer/20("rhoeps ")
  Reshape5/1 -> optimizer/19("duwt ")
  Reshape4/1 -> optimizer/18("uwt ")
  Reshape3/1 -> optimizer/17("ywt ")
  uref_scale/1 -> optimizer/16("MVtarget ")
  ext.mv_scale/1 -> optimizer/15("ext_mv ")
  Data Type Conversion8/1 -> optimizer/14("switch_in ")
  Reshape2/1 -> optimizer/13("S ")
  G Conversion/1 -> optimizer/12("G ")
  Reshape1/1 -> optimizer/11("F ")
  Reshape/1 -> optimizer/10("E ")
  ymax_scale/1 -> optimizer/9("ymax ")
  ymin_scale/1 -> optimizer/8("ymin ")
  umax_scale/1 -> optimizer/7("umax ")
  umin_scale/1 -> optimizer/6("umin ")
  Data Type Conversion2/1 -> optimizer/5("md ")
  Data Type Conversion1/1 -> optimizer/4("ref ")
  mo or x Conversion/1 -> optimizer/3("ym ")
  last_mv/1 -> optimizer/2("old_u ")
  last_x/1 -> optimizer/1("xk ")
  useq_scale1/1 -> y.seq/1
  Math Function2/1 -> Reshape5/1
  Math Function1/1 -> Reshape4/1
  Math Function/1 -> Reshape3/1
  MPC Matrix Signal Check1/1 -> F Conversion/1
  umin_scale4/1 -> Reshape/1
  ymin_scale1/1 -> Reshape1/1
  G/1 -> MPC Vector Signal Check1/1
  F/1 -> MPC Matrix Signal Check1/1
  E Conversion/1 -> umin_scale4/1
  ymin_scale2/1 -> Reshape2/1
  MPC Matrix Signal Check/1 -> E Conversion/1
  S/1 -> MPC Matrix Signal Check2/1
  E/1 -> MPC Matrix Signal Check/1
  MPC Matrix Signal Check2/1 -> S Conversion/1
  MPC Vector Signal Check1/1 -> G Conversion/1
  S Conversion/1 -> ymin_scale2/1
  F Conversion/1 -> ymin_scale1/1
  MPC Matrix Signal Check DX/1 -> Data Type Conversion21/1
  MPC Matrix Signal Check X/1 -> Data Type Conversion20/1
  MPC Matrix Signal Check Y/1 -> Data Type Conversion19/1
  MPC Matrix Signal Check U/1 -> Data Type Conversion18/1
  MPC Matrix Signal Check D/1 -> Data Type Conversion17/1
  MPC Matrix Signal Check C/1 -> Data Type Conversion16/1
  MPC Matrix Signal Check B/1 -> Data Type Conversion15/1
  MPC Matrix Signal Check A/1 -> Data Type Conversion14/1
  MPC Scalar Signal Check1/1 -> Data Type Conversion11/1
  MPC Preview Signal Check4/1 -> Data Type Conversion12/1
  MPC Preview Signal Check3/1 -> Data Type Conversion10/1
  MPC Preview Signal Check2/1 -> Data Type Conversion9/1
  MPC Vector Signal Check6/1 -> Data Type Conversion13/1
  MPC Vector Signal Check/1 -> Data Type Conversion3/1
  MPC Scalar Signal Check/1 -> Data Type Conversion8/1
  MPC Vector Signal Check2/1 -> Data Type Conversion7/1
  MPC Vector Signal Check3/1 -> Data Type Conversion6/1
  MPC Vector Signal Check4/1 -> Data Type Conversion5/1
  MPC Vector Signal Check5/1 -> Data Type Conversion4/1
  MPC Preview Signal Check1/1 -> Data Type Conversion2/1
  MPC Preview Signal Check/1 -> Data Type Conversion1/1
  MPC Vector Signal Check11/1 -> mo or x Conversion/1
  useq_scale/1 -> mv.seq/1
  u_scale/1 -> mv/1
  DX/1 -> MPC Matrix Signal Check DX/1
  X/1 -> MPC Matrix Signal Check X/1
  Y/1 -> MPC Matrix Signal Check Y/1
  U/1 -> MPC Matrix Signal Check U/1
  D/1 -> MPC Matrix Signal Check D/1
  C/1 -> MPC Matrix Signal Check C/1
  B/1 -> MPC Matrix Signal Check B/1
  A/1 -> MPC Matrix Signal Check A/1
  md/1 -> MPC Preview Signal Check1/1
  umin/1 -> MPC Vector Signal Check5/1
  umax/1 -> MPC Vector Signal Check4/1
  ymin/1 -> MPC Vector Signal Check3/1
  ymax/1 -> MPC Vector Signal Check2/1
  switch/1 -> MPC Scalar Signal Check/1
  ext.mv/1 -> MPC Vector Signal Check/1
  Data Type Conversion3/1 -> ext.mv_scale/1
  ref/1 -> MPC Preview Signal Check/1
  mo or x/1 -> MPC Vector Signal Check11/1
  ywt/1 -> MPC Preview Signal Check2/1
  uwt/1 -> MPC Preview Signal Check3/1
  Data Type Conversion4/1 -> umin_scale/1
  Data Type Conversion5/1 -> umax_scale/1
  Data Type Conversion7/1 -> ymax_scale/1
  Data Type Conversion9/1 -> Math Function/1
  Data Type Conversion12/1 -> Math Function2/1
  Data Type Conversion6/1 -> ymin_scale/1
  rhoeps/1 -> MPC Scalar Signal Check1/1
  duwt/1 -> MPC Preview Signal Check4/1
  Data Type Conversion10/1 -> Math Function1/1
  uref/1 -> MPC Vector Signal Check6/1
  Data Type Conversion13/1 -> uref_scale/1
  ym_zero/1 -> x_terminator/1

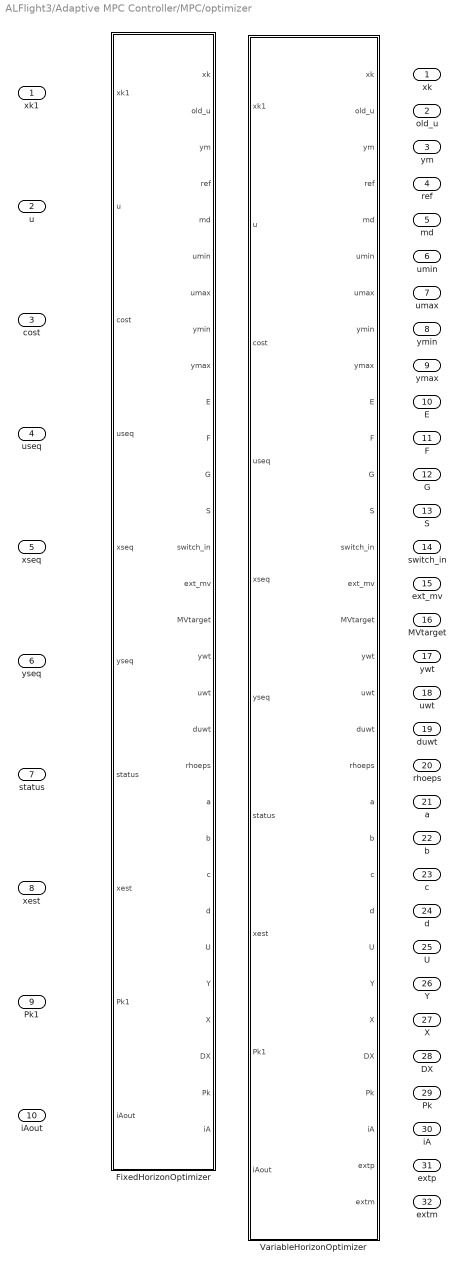
== system ALFlight3/Adaptive MPC Controller/MPC/optimizer ==
  "xk " : Inport
  "old_u " : Inport  Port=2
  "ym " : Inport  Port=3
  "ref " : Inport  Port=4
  "md " : Inport  Port=5
  "umin " : Inport  Port=6
  "umax " : Inport  Port=7
  "ymin " : Inport  Port=8
  "ymax " : Inport  Port=9
  "E " : Inport  Port=10
  "F " : Inport  Port=11
  "G " : Inport  Port=12
  "S " : Inport  Port=13
  "switch_in " : Inport  Port=14
  "ext_mv " : Inport  Port=15
  "MVtarget " : Inport  Port=16
  "ywt " : Inport  Port=17
  "uwt " : Inport  Port=18
  "duwt " : Inport  Port=19
  "rhoeps " : Inport  Port=20
  "a " : Inport  Port=21
  "b " : Inport  Port=22
  "c " : Inport  Port=23
  "d " : Inport  Port=24
  "U " : Inport  Port=25
  "Y " : Inport  Port=26
  "X " : Inport  Port=27
  "DX " : Inport  Port=28
  "Pk " : Inport  Port=29
  "iA " : Inport  Port=30
  extp : Inport  Port=31
  extm : Inport  Port=32
  FixedHorizonOptimizer : MATLAB Function  VariantControl=FixedHorizon
  VariableHorizonOptimizer : MATLAB Function  VariantControl=VariableHorizon
  " xk1" : Outport
  " u" : Outport  Port=2
  " cost" : Outport  Port=3
  " useq" : Outport  Port=4
  " xseq" : Outport  Port=5
  " yseq" : Outport  Port=6
  " status" : Outport  Port=7
  " xest" : Outport  Port=8
  " Pk1" : Outport  Port=9
  " iAout" : Outport  Port=10

== matlab function ALFlight3/MATLAB Function1 ==
  data: bestA output; uncertainty data_store_memory; savedInputs data_store_memory; savedOutputs data_store_memory; counts data_store_memory; currentState data_store_memory; in input; action data_store_memory; ABestGuess data_store_memory
function bestA= fcn10(in)
         coder.extrinsic('calcDynamics')
         coder.extrinsic('selectBayesianA')
global uncertainty
global savedInputs
global savedOutputs
global counts
global currentState
global action
global ABestGuess
coder.extrinsic('assignin')
    bestA=zeros(4,1);
    numStates=11;
    numOutputs=11;
    if counts>3
        inputsT=savedInputs(:,1:counts)
        outputsT=savedOutputs(:,1:counts)
        deltaSEst=zeros(numOutputs,counts);
        states=inputsT(5:15,:)
        actions=inputsT(1:4,:)

        for i =1:size(inputsT,2)
            deltaSEst(:,i)=simulateNominal(states(:,i),actions(:,i));
        end

        trainingInputs=[actions;deltaSEst];
        trainingOutputs=(outputsT-inputsT(5:end,:))/.05
           A=trainingInputs'\trainingOutputs'
           A=reshape(A,15,11)
        ABestGuess=A
        assignin('base','ABestGuess',ABestGuess)
        %%create bootstrapped models
        Z=4;
        NET = cell(Z,1);

        for i=1:size(NET,1)
            %indices of samples used for bootstrapping. Randomly sampled with replacement
            bootSamples= randi(size(trainingInputs,2),size(trainingInputs,2),1);
            xBoot=zeros(15,counts);
            yBoot=zeros(11,counts);
            %Pick out samples from training inputs and outputs
            for b=1:size(trainingInputs,2)
                xBoot(:,b)=trainingInputs(:,bootSamples(b));
                yBoot(:,b)=trainingOutputs(:,bootSamples(b));
            end
            %All samples used for trainging and testing
            NET{i}=xBoot'\yBoot';
            %uncertainty=uncertainty+sum(sum(abs(ABestGuess-NET{i})))
 
        end

        %find best action subject to constraints
%         A = [];
%         b = [];
%         Aeq = [];
%         beq = [];
%         lb = [-30,35000,-30,-30];
%         ub = [30,70000,30,30];
%         nonlcon=[];
%         IntCon=[];
%         options = optimoptions('ga','FitnessLimit', 17);
%         options = optimoptions('ga','Generations', 10);
%         options = optimoptions('ga','TimeLimit', 20);

        %bestA=patternsearch(@findBestA,[0 5.5e5 0 0],A,b,Aeq,beq,lb,ub,@setUpConstraints);
%         uncertainty=evalin('base','uncertainty')
%         if uncertainty>100
%             bestA=ga(@findBestA,4,A,b,Aeq,beq,lb,ub,[],options)
%         else
%             bestA=ga(@findBestA,4,A,b,Aeq,beq,lb,ub,@setUpConstraints,options);
%         end
%         bestA=bestA';
       tic
         [bestA,u]=selectRandomA(currentState,uncertainty,ABestGuess,NET,action)

         %ABestGuess=calcDynamics(trainingInputs,trainingOutputs)
        
         %[bestA,u]=selectBayesianA(currentState,uncertainty,action,ABestGuess,trainingInputs,trainingOutputs)
         uncertainty=u
         %assignin('base','toc2',toc)
%         
%     end
    
%     function a=selectRandomA(currentState)
%         num=200
%         currentState=evalin('base','currentState')
%         elevator=(30+30).*rand(1,num)-30;
%         thrust=(20000).*rand(1,num)+40000;
%         aileron=(30+30).*rand(1,num)-30;
%         rudder=(30+30).*rand(1,num)-30;
%         actionsTest=[elevator;thrust;aileron;rudder]
%         posInput=[];
%        counter=0
%        uncertainty=evalin('base','uncertainty')
%        goal=[40,10,-50]
%        if uncertainty<100
%            goal=goal*(uncertainty/100)^.5
%            assignin('base','goal',goal)
%             for k=1:num
%                 stateEst3=simulateNominal(currentState,actionsTest(:,k));
%                 y=sim(netFail2Simulink,[actionsTest(:,k);stateEst3])
%                 if y(1,1)<160+goal(1) && y(1,1)>160-goal(1) && abs(y(4,1))<goal(2) && abs(y(8,1))<goal(2) && abs(y(9,1))<goal(2) && y(11,1)>goal(3)
%                     posInput=[posInput actionsTest(:,k)];
%                     counter=counter+1
%                     assignin('base','y',y)
%                 end
%             end
%        end
%         assignin('base','counter',counter)
%         nmax=0;
%         index=1;
%         if isempty(posInput)
%             posInput=actionsTest
%         end
%         assignin('base','posInput',posInput)
%         for pos=1:size(posInput,2)
%             currentState=evalin('base','currentState');    
%             stateEst2=simulateNominal(currentState,posInput(:,pos));
%             y=sim(netFail2Simulink,[posInput(:,pos);stateEst2]);
%             n=0;
%             for j=1:size(NET,1)       
%                 yZ=sim(NET{j},[posInput(:,pos);stateEst2]);
%                 %n=n+norm(defaultderiv('dperf_dwb',netFail2,[input(1:4);stateEst2],yZ));
%                 %n=n+norm(sum(y-yZ)*input,1); 
%                 n=sum(abs(y-yZ)); 
%             end
%             nFinal=n/4.0;
%             if nFinal>nmax
%                 nmax=nFinal;
%                 index=pos
% 
%             end
%             
%         end
%         max2=evalin('base','max2')
%         assignin('base','max2',[max2 nmax])
%         assignin('base','uncertainty',nmax)
%         a=posInput(:,index)
%         
%     end
%         
% 
% 
%     
%     
%     function nFinal=findBestA(safeAction)
%         safeAction=safeAction';
%         currentState=evalin('base','currentState');    
%         stateEst2=simulateNominal(currentState,safeAction);
%         y=sim(netFail2Simulink,[safeAction;stateEst2]);
%         n=0;
%         for j=1:size(NET,1)       
%             yZ=sim(NET{j},[safeAction;stateEst2]);
%             %n=n+norm(defaultderiv('dperf_dwb',netFail2,[input(1:4);stateEst2],yZ));
%             %n=n+norm(sum(y-yZ)*input,1); 
%             n=sum(abs(y-yZ)); 
%         end
%         nFinal=-n/4.0;
%         assignin('base','uncertainty',nFinal*(-1))
%         assignin('base','y1',y)
%     end

end






% time=input(1)
% if time>2.8
% savedInputs=evalin('base','savedInputs')
% savedOutputs=evalin('base','savedOutputs')
% action=input(2:5);
% state=input(6:16);
% output=input(17:27);
% 
% stateEst=simulateNominal(state,action);
% trainingIn=[[action;stateEst],savedInputs];
% size(trainingIn)
% trainingOut=[output,savedOutputs];
% assignin('base','savedInputs',trainingIn)
% assignin('base','savedOutputs',trainingOut)
% 
% hiddenLayerSize = [10];
% netFail2SimulinkUpdate = fitnet(hiddenLayerSize)
% netFail2SimulinkUpdate.trainParam.epochs = 10
% netFail2SimulinkUpdate.layers{1}.transferFcn = 'purelin';
% netFail2SimulinkUpdate.divideFcn = 'divideind';
% netFail2SimulinkUpdate.divideParam.trainInd = 1:16;
% netFail2SimulinkUpdate.divideParam.valInd = [];
% netFail2SimulinkUpdate.divideParam.testInd = [];
%  %Train the Network
% [netFail2SimulinkUpdate,trFail2] = train(netFail2SimulinkUpdate,trainingIn,trainingOut);
%end
